simulink model "zad1model23456"  (R2024a)
settings: Solver=VariableStepAuto  StartTime=0.0  StopTime=10.0  RelTol=1e-3
settings Model: Creator=adasf  LastModifiedBy=adasf

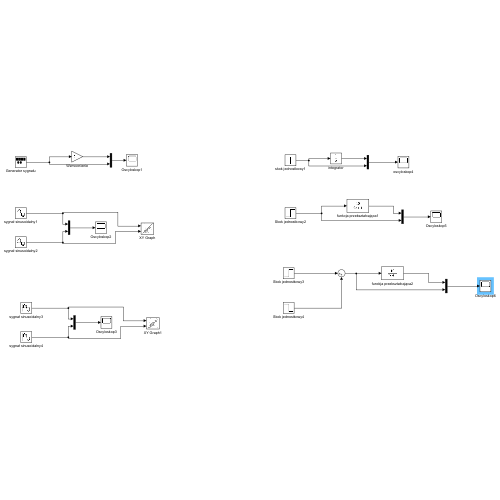
[thumbnail: Simulink's stored preview of the top-level diagram]
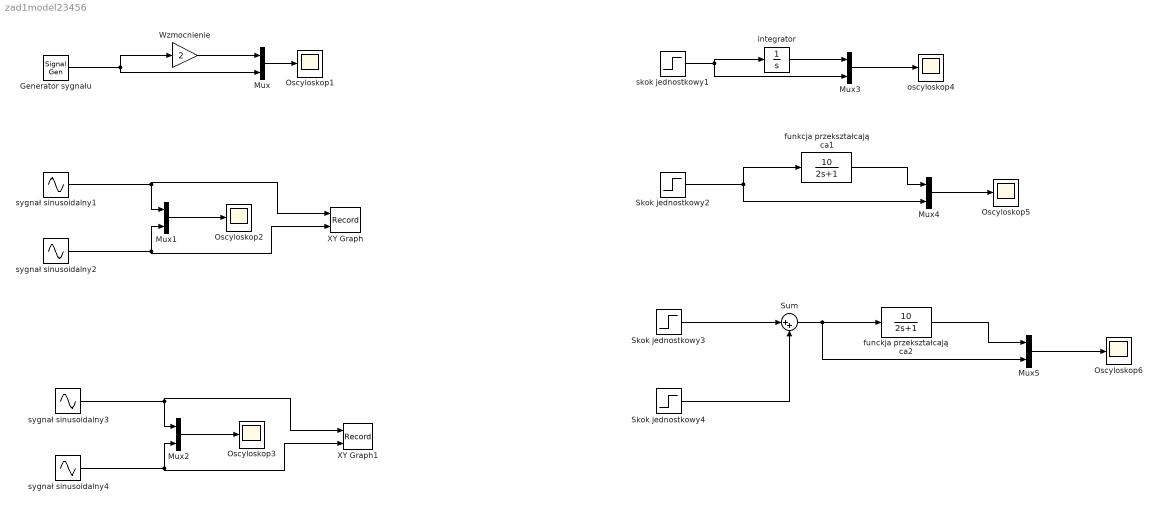
== system zad1model23456 ==
  Generator sygnału : SignalGenerator  Units=rad/sec
  Mux{,1..5} (6 alike) : Mux  Inputs=2
  Oscyloskop{1..3,5..6} (5 alike) : Scope
  Skok jednostkowy2 : Step  After=5  SampleTime=0
  Skok jednostkowy3 : Step  Time=0  After=10  SampleTime=0
  Skok jednostkowy4 : Step  Time=0.1  After=-10  SampleTime=0
  Sum : Sum  Inputs=|++
  Wzmocnienie : Gain  Gain=2
  XY Graph : Record  FileSettingsInternal="{\"entries\":[{\"content\":{\"excelSettings\":{\"content\":{},\"type\":\"Streamout.ExcelSettings\"}},\"type\":\"Streamout.FileSettingStorage\",\"uuid\":\"\"}],\"packageUris\":[\"http:\\/\\/schema.mathworks.com\\/mf0\\/streamout_blocks\\/R2020a\"],\"version\":\"1.0\"}"  Layout=[1 1]  SignalsInternal="{\"entries\":[{\"content\":{\"signals\":[{\"content\":{\"blockPath\":[],\"dimensions\":[1],\"domain\":\"\",\"lineColor\":\"#a2142f\",\"plots\":[ 1 ],\"port\":1,\"sid\":[\"\"],\"signalID\":1,\"signalName\":\"sygnał sinusoidalny1\"},\"type\":\"RecordBlkView.Signal\",\"uuid\":\"\"},{\"content\":{\"blockPath\":[],\"dimensions\":[1],\"domain\":\"\",\"lineColor\":\"#139fff\",\"plots\":[ 1 ],\"port\":2,\"sid\":[\"\"],\"signalID\":2,\"signalName\":\"sygnał sinusoidalny2\"},\"type\":\"RecordBlkView.Signal\",\"uuid\":\"\"}]},\"type\":\"RecordBlkView.InputSignals\",\"uuid\":\"\"}],\"packageUris\":[\"http:\\/\\/schema.mathworks.com\\/mf0\\/streamout_blocks\\/R2020a\"],\"version\":\"1.0\"}"  VisualizationBindings="{\"xyplotplugin\":{\"info\":[{\"series\":[{\"bindingParametersList\":[{\"parameter\":\"X-Axis\",\"signalID\":1,\"signalName\":\"sygnał sinusoidalny1\"},{\"parameter\":\"Y-Axis\",\"signalID\":2,\"signalName\":\"sygnał sinusoidalny2\"}],\"seriesID\":0}],\"subplotID\":1}]}}"  CompatibilityTag=XY
  XY Graph1 : Record  FileSettingsInternal="{\"entries\":[{\"content\":{\"excelSettings\":{\"content\":{},\"type\":\"Streamout.ExcelSettings\"}},\"type\":\"Streamout.FileSettingStorage\",\"uuid\":\"\"}],\"packageUris\":[\"http:\\/\\/schema.mathworks.com\\/mf0\\/streamout_blocks\\/R2020a\"],\"version\":\"1.0\"}"  Layout=[1 1]  SignalsInternal="{\"entries\":[{\"content\":{\"signals\":[{\"content\":{\"blockPath\":[],\"dimensions\":[1],\"domain\":\"\",\"lineColor\":\"#a2142f\",\"plots\":[ 1 ],\"port\":1,\"sid\":[\"\"],\"signalID\":1,\"signalName\":\"sygnał sinusoidalny3\"},\"type\":\"RecordBlkView.Signal\",\"uuid\":\"\"},{\"content\":{\"blockPath\":[],\"dimensions\":[1],\"domain\":\"\",\"lineColor\":\"#139fff\",\"plots\":[ 1 ],\"port\":2,\"sid\":[\"\"],\"signalID\":2,\"signalName\":\"sygnał sinusoidalny4\"},\"type\":\"RecordBlkView.Signal\",\"uuid\":\"\"}]},\"type\":\"RecordBlkView.InputSignals\",\"uuid\":\"\"}],\"packageUris\":[\"http:\\/\\/schema.mathworks.com\\/mf0\\/streamout_blocks\\/R2020a\"],\"version\":\"1.0\"}"  VisualizationBindings="{\"xyplotplugin\":{\"info\":[{\"series\":[{\"bindingParametersList\":[{\"parameter\":\"X-Axis\",\"signalID\":1,\"signalName\":\"sygnał sinusoidalny3\"},{\"parameter\":\"Y-Axis\",\"signalID\":2,\"signalName\":\"sygnał sinusoidalny4\"}],\"seriesID\":0}],\"subplotID\":1}]}}"  CompatibilityTag=XY
  funckja przekształcająca2 : TransferFcn  Numerator=[10]  Denominator=[2 1]
  funkcja przekształcająca1 : TransferFcn  Numerator=[10]  Denominator=[2 1]
  integrator : Integrator
  oscyloskop4 : Scope
  skok jednostkowy1 : Step  After=5  SampleTime=0
  sygnał sinusoidalny1 : Sin  Amplitude=5  Frequency=3  Phase=pi / 2  SampleTime=0.01
  sygnał sinusoidalny2 : Sin  Amplitude=5  Frequency=2  SampleTime=0.01
  sygnał sinusoidalny3 : Sin  Amplitude=5  Frequency=3  Phase=pi / 2  SampleTime=0.01
  sygnał sinusoidalny4 : Sin  Amplitude=5  Frequency=2  SampleTime=0.01
  wires:
  Mux/1 -> Oscyloskop1/1
  Generator sygnału/1 -> Mux/2, Wzmocnienie/1
  Wzmocnienie/1 -> Mux/1
  sygnał sinusoidalny2/1 -> Mux1/2, XY Graph/2
  sygnał sinusoidalny1/1 -> Mux1/1, XY Graph/1
  Mux1/1 -> Oscyloskop2/1
  Mux2/1 -> Oscyloskop3/1
  sygnał sinusoidalny3/1 -> Mux2/1, XY Graph1/1
  sygnał sinusoidalny4/1 -> Mux2/2, XY Graph1/2
  skok jednostkowy1/1 -> integrator/1, Mux3/2
  integrator/1 -> Mux3/1
  Mux3/1 -> oscyloskop4/1
  Skok jednostkowy2/1 -> Mux4/2, funkcja przekształcająca1/1
  funkcja przekształcająca1/1 -> Mux4/1
  Mux4/1 -> Oscyloskop5/1
  Skok jednostkowy3/1 -> Sum/1
  Skok jednostkowy4/1 -> Sum/2
  Sum/1 -> Mux5/2, funckja przekształcająca2/1
  funckja przekształcająca2/1 -> Mux5/1
  Mux5/1 -> Oscyloskop6/1
